simulink model "proba1"  (Simulink 7.0)
settings: Solver=ode1  StartTime=0.0  StopTime=Inf  FixedStep=0.001  RelTol=1e-3
PostLoadFcn:
  | ,try, rti_mdl_postloadfcn(bdroot, 'UpdateModel', 280, 'rti1005'); catch, disp(lasterr); end,
values from neighbouring files (symbols this model uses):
  Rmax = 823    [50614_11.mat]    (also in 50614_7.mat)
  Rmin = 331    [50614_11.mat]    (also in 50614_7.mat)
undefined symbols (not defined in the file or in its folder): sgn
libraries: simulink x68, simulink_extras x15, rtilibm x10
(part 3 of 3)

== system proba1/tryby/rozpoznawanie obrazu/optymalizacja1/warunek na Fi/Subsystem1 ==
  In1 : Inport
  Add : Sum  Inputs=++|
  Data Store Read6 : DataStoreRead  DataStoreName=yKon  SampleTime=-1
  Logical Operator4 : Logic  AllPortsSameDT=off  OutDataTypeMode=boolean
  do Xmax : simulink/Logic and Bit Operations/Compare To Constant  SystemSampleTime=-1  relop=<  const=1600  LogicOutDataTypeMode=uint8  ZeroCross=off
  do Xmin : simulink/Logic and Bit Operations/Compare To Constant  SystemSampleTime=-1  relop=>  const=0  LogicOutDataTypeMode=uint8  ZeroCross=off
  Out1 : Outport
  wires:
  Data Store Read6/1 -> Add/2
  do Xmin/1 -> Logical Operator4/1
  do Xmax/1 -> Logical Operator4/2
  Add/1 -> do Xmin/1, do Xmax/1
  Logical Operator4/1 -> Out1/1
  In1/1 -> Add/1

== system proba1/tryby/rozpoznawanie obrazu/optymalizacja1/warunek na Fi/Subsystem4 ==
  In1 : Inport
  Add : Sum  Inputs=++|
  Data Store Read6 : DataStoreRead  DataStoreName=yKon  SampleTime=-1
  Logical Operator4 : Logic  AllPortsSameDT=off  OutDataTypeMode=boolean
  do Xmax : simulink/Logic and Bit Operations/Compare To Constant  SystemSampleTime=-1  relop=<  const=1600  LogicOutDataTypeMode=uint8  ZeroCross=off
  do Xmin : simulink/Logic and Bit Operations/Compare To Constant  SystemSampleTime=-1  relop=>  const=0  LogicOutDataTypeMode=uint8  ZeroCross=off
  Out1 : Outport
  wires:
  In1/1 -> Add/1
  Logical Operator4/1 -> Out1/1
  Add/1 -> do Xmax/1, do Xmin/1
  Data Store Read6/1 -> Add/2
  do Xmax/1 -> Logical Operator4/2
  do Xmin/1 -> Logical Operator4/1

== system proba1/tryby/rozpoznawanie obrazu/optymalizacja1/warunek na R/Subsystem1 ==
  In1 : Inport
  Add : Sum  Inputs=++|
  Data Store Read6 : DataStoreRead  DataStoreName=yKon  SampleTime=-1
  Logical Operator4 : Logic  AllPortsSameDT=off  OutDataTypeMode=boolean
  do Xmax : simulink/Logic and Bit Operations/Compare To Constant  SystemSampleTime=-1  relop=<  const=1600  LogicOutDataTypeMode=uint8  ZeroCross=off
  do Xmin : simulink/Logic and Bit Operations/Compare To Constant  SystemSampleTime=-1  relop=>  const=0  LogicOutDataTypeMode=uint8  ZeroCross=off
  Out1 : Outport
  wires:
  Data Store Read6/1 -> Add/2
  do Xmin/1 -> Logical Operator4/1
  do Xmax/1 -> Logical Operator4/2
  Add/1 -> do Xmin/1, do Xmax/1
  Logical Operator4/1 -> Out1/1
  In1/1 -> Add/1

== system proba1/tryby/rozpoznawanie obrazu/optymalizacja1/warunek na R/Subsystem2 ==
  In2 : Inport
  In3 : Inport  Port=2
  Demux : Demux  Outputs=2
  Gain : Gain  Gain=-1
  Logical Operator1 : Logic  AllPortsSameDT=off  OutDataTypeMode=boolean
  Mux3 : Mux  Inputs=2
  Terminator : Terminator
  Xgran : Fcn  Expr=u(1)*sin(u(2))
  Xgran1 : Fcn  Expr=u(4)-u(2)
  do Fimax : simulink/Logic and Bit Operations/Compare To Constant  SystemSampleTime=-1  relop=<=  const=2.792527  LogicOutDataTypeMode=uint8  ZeroCross=off
  do Fimin : simulink/Logic and Bit Operations/Compare To Constant  SystemSampleTime=-1  relop=>=  const=-2.792527  LogicOutDataTypeMode=uint8  ZeroCross=off
  Out1 : Outport
  Out2 : Outport  Port=2
  wires:
  Gain/1 -> Out1/1
  Xgran1/1 -> Gain/1
  Demux/1 -> Terminator/1
  Demux/2 -> do Fimax/1, do Fimin/1
  Logical Operator1/1 -> Out2/1
  In3/1 -> Demux/1, Xgran/1
  In2/1 -> Mux3/1
  Mux3/1 -> Xgran1/1
  Xgran/1 -> Mux3/2
  do Fimax/1 -> Logical Operator1/1
  do Fimin/1 -> Logical Operator1/2

== system proba1/tryby/rozpoznawanie obrazu/optymalizacja1/warunek na R/Subsystem3 ==
  In2 : Inport
  In3 : Inport  Port=2
  Demux : Demux  Outputs=2
  Gain : Gain  Gain=-1
  Logical Operator1 : Logic  AllPortsSameDT=off  OutDataTypeMode=boolean
  Mux3 : Mux  Inputs=2
  Terminator : Terminator
  Xgran : Fcn  Expr=-u(1)*sin(u(2))
  Xgran1 : Fcn  Expr=u(4)-u(2)
  do Fimax : simulink/Logic and Bit Operations/Compare To Constant  SystemSampleTime=-1  relop=<=  const=2.792527  LogicOutDataTypeMode=uint8  ZeroCross=off
  do Fimin : simulink/Logic and Bit Operations/Compare To Constant  SystemSampleTime=-1  relop=>=  const=-2.792527  LogicOutDataTypeMode=uint8  ZeroCross=off
  Out1 : Outport
  Out2 : Outport  Port=2
  wires:
  Gain/1 -> Out1/1
  Demux/1 -> Terminator/1
  Demux/2 -> do Fimax/1, do Fimin/1
  do Fimin/1 -> Logical Operator1/2
  do Fimax/1 -> Logical Operator1/1
  Xgran/1 -> Mux3/2
  Xgran1/1 -> Gain/1
  Mux3/1 -> Xgran1/1
  In2/1 -> Mux3/1
  In3/1 -> Xgran/1, Demux/1
  Logical Operator1/1 -> Out2/1

== system proba1/tryby/rozpoznawanie obrazu/optymalizacja1/warunek na R/Subsystem4 ==
  In1 : Inport
  Add : Sum  Inputs=++|
  Data Store Read6 : DataStoreRead  DataStoreName=yKon  SampleTime=-1
  Logical Operator4 : Logic  AllPortsSameDT=off  OutDataTypeMode=boolean
  do Xmax : simulink/Logic and Bit Operations/Compare To Constant  SystemSampleTime=-1  relop=<  const=1600  LogicOutDataTypeMode=uint8  ZeroCross=off
  do Xmin : simulink/Logic and Bit Operations/Compare To Constant  SystemSampleTime=-1  relop=>  const=0  LogicOutDataTypeMode=uint8  ZeroCross=off
  Out1 : Outport
  wires:
  In1/1 -> Add/1
  Logical Operator4/1 -> Out1/1
  Add/1 -> do Xmax/1, do Xmin/1
  Data Store Read6/1 -> Add/2
  do Xmax/1 -> Logical Operator4/2
  do Xmin/1 -> Logical Operator4/1
